simulink model "Furnace"  (R2020a)
settings: Solver=ode15s  StartTime=0  StopTime=12000  FixedStep=0.1  MaxStep=20  RelTol=1e-08  AbsTol=1e-09
undefined symbols (not defined in the file): k, reg
libraries: simulink x9, mpclib x1
(part 1 of 3)
settings Model: SimulationMode=accelerator  Creator=elisam  LastModifiedBy=jorn
settings SolverCC: MaxConsecutiveZCs=10000  ZeroCrossAlgorithm=Adaptive
settings DataIOCC: FinalStateName=ss_state_out  InitialState=ss_state  SaveFinalState=on  SaveOperatingPoint=on  SaveFormat=StructureWithTime  SaveOutput=off  DSMLogging=off  ReturnWorkspaceOutputs=off
settings OptimizationCC: BlockReduction=off  EfficientMapNaN2IntZero=off  SimCompilerOptimization=on
settings DebuggingCC: AlgebraicLoopMsg=error  ArtificialAlgebraicLoopMsg=error  UnconnectedInputMsg=none  UnconnectedOutputMsg=none  UnconnectedLineMsg=none  PregeneratedLibrarySubsystemCodeDiagnostic=none  ArithmeticOperatorsInVariantConditions=warning
settings HardwareCC: TargetBitPerLong=64  TargetBitPerPointer=64  TargetBitPerSizeT=64  TargetBitPerPtrDiffT=64  TargetLongLongMode=on  TargetIntDivRoundTo=Zero  TargetEndianess=LittleEndian  TargetWordSize=64  TargetHWDeviceType=MATLAB Host  ProdEqTarget=off
settings SFSimCC: SimUseLocalCustomCode=off  CustomCodeUndefinedFunction=UseInterfaceOnly
settings CodeAppCC: MaxIdLength=128
settings GRTTargetCC: TargetLangStandard=C89/C90 (ANSI)  CombineOutputUpdateFcns=off  GRTInterface=on

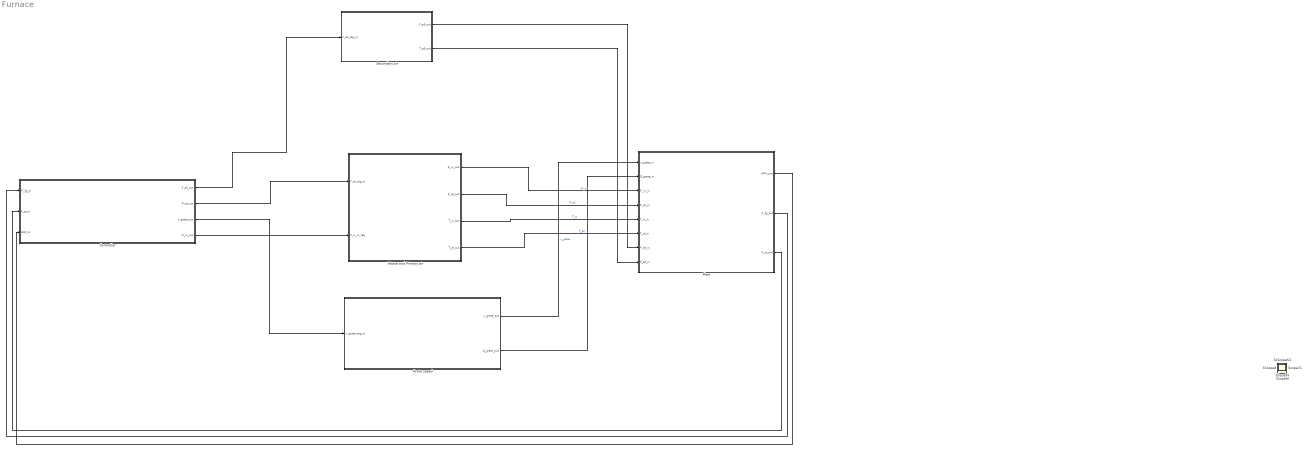
== system Furnace ==
  Controller : Subsystem
  Grate speed : Subsystem
  Plant : Subsystem
  Secondary air : Subsystem
      mask Display: image('airflow.jpeg');
  Waste and Primary air : Subsystem
      mask Display: image('waste_in.jpg');
  Scope{,1..15,17..21} (21 alike) : Scope
  wires:
  Controller/1(F_aII_out) -> Secondary air/1(F_aII_reg_in)
  Controller/2(Fi_aI_out) -> Waste and Primary air/1("F_aI_reg_in ")
  Controller/3(v_grate_out) -> Grate speed/1(v_grate_reg_in)
  Controller/4(Fi_w_out) -> Waste and Primary air/2(F_w_in_reg)
  Grate speed/1(v_grate_out) -> Plant/1(v_grate_in)  "v_grate"
  Grate speed/2(Q_grate_out) -> Plant/2(Q_grate_in)
  Plant/2(F_fg_out) -> Controller/1(Fi_fg_in)
  Plant/3(F_st_out) -> Controller/2(F_st_in)
  Waste and Primary air/1(Fi_w_out) -> Plant/3(Fi_w_in)  "Fi_w"
  Waste and Primary air/2(Fi_aI_out) -> Plant/4(Fi_aI_in)  "Fi_aI"
  Waste and Primary air/3(T_w_out) -> Plant/5(T_w_in)  "T_w"
  Waste and Primary air/4(T_aI_out) -> Plant/6(T_aI_in)  "T_aI"
  Secondary air/1(F_aII_out) -> Plant/7(F_aII_in)
  Secondary air/2(T_aII_out) -> Plant/8(T_aII_in)
  Plant/1(HHV_out) -> Controller/3(HHV_in)

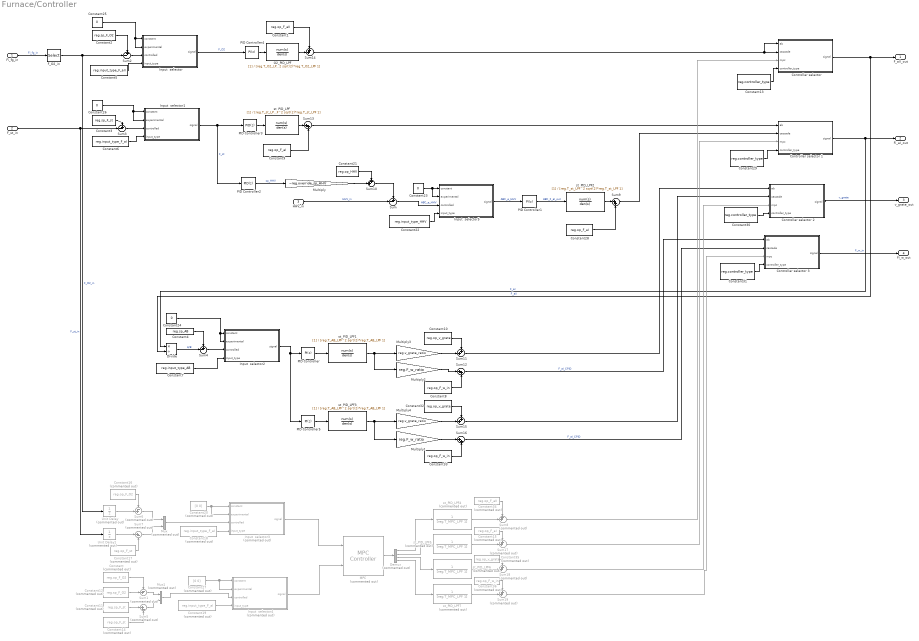
== system Furnace/Controller ==
  Fi_fg_in : Inport
  F_st_in : Inport  Port=2
  HHV_in : Inport  Port=3
  Constant : Constant  Commented=on  Value=reg.op_F_O2
  Constant1 : Constant  Value=reg.op_F_aII
  Constant10 : Constant  Value=reg.op_v_grate
  Constant11 : Constant  Commented=on  Value=reg.sp_F_st
  Constant12 : Constant  Commented=on  Value=reg.sp_F_O2
  Constant{13,29..31} (4 alike) : Constant  Value=reg.controller_type
  Constant14 : Constant  Commented=on  Value=reg.op_F_st
  Constant15 : Constant  Commented=on  Value=reg.op_F_aI
  Constant16 : Constant  Commented=on  Value=reg.op_F_O2
  Constant17 : Constant  Commented=on  Value=reg.op_F_st
  Constant18 : Constant  Commented=on  Value=reg.input_type_F_aI
  Constant19 : Constant  Commented=on  Value=reg.input_type_F_aI
  Constant2 : Constant  Value=reg.sp_F_O2
  Constant20 : Constant  Commented=on  Value=[0 0]
  Constant21 : Constant  Value=reg.op_HHV
  Constant22 : Constant  Value=reg.input_type_HHV
  Constant{23..26} (4 alike) : Constant  Value=0
  Constant27 : Constant  Commented=on  Value=[0 0]
  Constant28 : Constant  Value=reg.op_F_aI
  Constant3 : Constant  Value=reg.sp_F_st
  Constant32 : Constant  Value=reg.op_v_grate
  Constant33 : Constant  Value=reg.op_F_w_in
  Constant34 : Constant  Commented=on  Value=reg.op_F_aII
  Constant35 : Constant  Commented=on  Value=reg.op_v_grate
  Constant36 : Constant  Commented=on  Value=reg.op_F_w_in
  Constant4 : Constant  Value=reg.sp_AB
  Constant5 : Constant  Value=reg.input_type_F_aII
  Constant6 : Constant  Value=reg.input_type_F_aI
  Constant7 : Constant  Value=reg.input_type_AB
  Constant8 : Constant  Value=reg.op_F_w_in
  Constant9 : Constant  Value=reg.op_F_aI
  "Controller selector " : MATLAB Function  TreatAsAtomicUnit=on
  Controller selector 1 : MATLAB Function  TreatAsAtomicUnit=on
  Controller selector 2 : MATLAB Function  TreatAsAtomicUnit=on
  Controller selector 3 : MATLAB Function  TreatAsAtomicUnit=on
  Demux : Demux  Commented=on
  Divide : Product  Inputs=*/  OutMin=[-100]  OutMax=[100]
  F_O2_in : Selector  InputPortWidth=12  IndexOptions=Index vector (dialog)  Indices=[4]  OutputSizes=1
  Input  selector : MATLAB Function  TreatAsAtomicUnit=on
  Input  selector1 : MATLAB Function  TreatAsAtomicUnit=on
  Input  selector2 : MATLAB Function  TreatAsAtomicUnit=on
  Input  selector3 : MATLAB Function  Commented=on  TreatAsAtomicUnit=on
  Input  selector4 : MATLAB Function  Commented=on  TreatAsAtomicUnit=on
  Input  selector5 : MATLAB Function  TreatAsAtomicUnit=on
  MPC : mpclib/MPC Controller  Commented=on  SCDEnableBlockLinearizationSpecification=on  mpcobj=lmpc  is_multiple=0  enable_value=0  return_u0=off  updateMPCinCallerWorkspace=on  md_inport=off  mv_inport=off  uref_inport=off  return_cost=off  return_mvseq=off  return_qpstatus=off  return_xseq=off  return_state=off  return_ovseq=off  state_inport=off  umin_inport=off  umax_inport=off  ymin_inport=off  ymax_inport=off  cc_inport=off  ywt_inport=off  uwt_inport=off  duwt_inport=off  rhoeps_inport=off  pm_inport=off  MaximumP=10  HorizonChoice=FixedHorizon  n_ts=20  n_p=50  n_mv=4  n_md=0  n_ud=0  n_mo=2  n_uo=0  BlockDataType=double  SampleTimeInherited=off  switch_inport=off
  Multiply : Gain  Gain=~reg.override_sp_HHV
  Multiply1 : Gain  Gain=reg.F_w_ratio
  Multiply2 : Gain  Gain=reg.F_w_ratio
  Multiply3 : Gain  Gain=reg.v_grate_ratio
  Multiply4 : Gain  Gain=reg.v_grate_ratio
  Mux : Mux  Commented=on  Inputs=2
  Mux1 : Mux  Commented=on  Inputs=2
  O2_PID_LPF : TransferFcn  Denominator=[reg.T_O2_LPF^2 sqrt(2)*reg.T_O2_LPF 1]
  PID Controller : simulink/Continuous/PID Controller  Controller=PI  Form=Parallel  TimeDomain=Discrete-time  UseExternalTs=off  SampleTime=1  IntegratorMethod=Forward Euler  FilterMethod=Forward Euler  ControllerParametersSource=internal  P=reg.Kp_AB  I=reg.Ki_AB  D=0  UseFilter=on  N=100  TunerSelectOption=Transfer Function Based (PID Tuner App)  InitialConditionSource=internal  InitialConditionForIntegrator=0  InitialConditionForFilter=0  DifferentiatorICPrevScaledInput=0  ExternalReset=none  TrackingMode=off  Kt=1  LimitOutput=off  UpperSaturationLimit=inf  LowerSaturationLimit=-inf  LinearizeAsGain=on  AntiWindupMode=none  Kb=1  POutMin=[]  POutMax=[]  IOutMin=[]  IOutMax=[]  DOutMin=[]  DOutMax=[]  NOutMin=[]  NOutMax=[]  SumOutMin=[]  SumOutMax=[]  SaturationOutMin=[]  SaturationOutMax=[]  PParamMin=[]  PParamMax=[]  IParamMin=[]  IParamMax=[]  DParamMin=[]  DParamMax=[]  NParamMin=[]  NParamMax=[]  KbParamMin=[]  KbParamMax=[]  KtParamMin=[]  KtParamMax=[]  KbOutMin=[]  KbOutMax=[]  KtOutMin=[]  KtOutMax=[]  IntegratorOutMin=[]  IntegratorOutMax=[]  FilterOutMin=[]  FilterOutMax=[]  SumI1OutMin=[]  SumI1OutMax=[]  SumI2OutMin=[]  SumI2OutMax=[]  SumI3OutMin=[]  SumI3OutMax=[]  SumI4OutMin=[]  SumI4OutMax=[]  SumDOutMin=[]  SumDOutMax=[]  DifferentiatorOutMin=[]  DifferentiatorOutMax=[]  FilterDiffOutCoefMin=[]  FilterDiffOutCoefMax=[]  ReciprocalOutMin=[]  ReciprocalOutMax=[]  SumDenOutMin=[]  SumDenOutMax=[]  SumNumOutMin=[]  SumNumOutMax=[]  DivideOutMin=[]  DivideOutMax=[]  UdiffTsProdOutMin=[]  UdiffTsProdOutMax=[]  NTsProdOutMin=[]  NTsProdOutMax=[]  UintegralTsProdOutMin=[]  UintegralTsProdOutMax=[]  UngainTsProdOutMin=[]  UngainTsProdOutMax=[]  IntegratorContinuousStateAttributes=''  IntegratorStateMustResolveToSignalObject=off  IntegratorRTWStateStorageClass=Auto  FilterContinuousStateAttributes=''  FilterStateMustResolveToSignalObject=off  FilterRTWStateStorageClass=Auto  ParallelPVariant=InternalParameters  IdealPVariant=Disabled  IVariant=InternalParameters  DVariant=Disabled  IntegratorVariant=Discrete  SatVariant=Disabled  AWVariant=Passthrough  PCopyVariant=Disabled  TRVariant=Disabled  FdbkBlocksVariant=Forward  IdealPFdbkVariant=Disabled  SatFdbkVariant=Disabled  DerivativeFilterVariant=Disabled  NVariant=Disabled  NCopyVariant=Disabled_SignalSpec  FilterICVariant=Disabled  IntegratorICVariant=InternalICs  ExternalResetVariant=Disabled  TRSumVariant=Passthrough  SumFdbkVariant=Disabled  SumVariant=Sum_PI  TsampFilterVariant=InternalTs  TsampNgainVariant=Passthrough  TsampIntegralVariant=Passthrough
  PID Controller1 : simulink/Continuous/PID Controller  Controller=PI  Form=Parallel  TimeDomain=Discrete-time  UseExternalTs=off  SampleTime=1  IntegratorMethod=Forward Euler  FilterMethod=Forward Euler  ControllerParametersSource=internal  P=reg.Kp_HHV  I=reg.Ki_HHV  D=0  UseFilter=on  N=100  TunerSelectOption=Transfer Function Based (PID Tuner App)  InitialConditionSource=internal  InitialConditionForIntegrator=0  InitialConditionForFilter=0  DifferentiatorICPrevScaledInput=0  ExternalReset=none  TrackingMode=off  Kt=1  LimitOutput=off  UpperSaturationLimit=inf  LowerSaturationLimit=-inf  LinearizeAsGain=on  AntiWindupMode=none  Kb=1  POutMin=[]  POutMax=[]  IOutMin=[]  IOutMax=[]  DOutMin=[]  DOutMax=[]  NOutMin=[]  NOutMax=[]  SumOutMin=[]  SumOutMax=[]  SaturationOutMin=[]  SaturationOutMax=[]  PParamMin=[]  PParamMax=[]  IParamMin=[]  IParamMax=[]  DParamMin=[]  DParamMax=[]  NParamMin=[]  NParamMax=[]  KbParamMin=[]  KbParamMax=[]  KtParamMin=[]  KtParamMax=[]  KbOutMin=[]  KbOutMax=[]  KtOutMin=[]  KtOutMax=[]  IntegratorOutMin=[]  IntegratorOutMax=[]  FilterOutMin=[]  FilterOutMax=[]  SumI1OutMin=[]  SumI1OutMax=[]  SumI2OutMin=[]  SumI2OutMax=[]  SumI3OutMin=[]  SumI3OutMax=[]  SumI4OutMin=[]  SumI4OutMax=[]  SumDOutMin=[]  SumDOutMax=[]  DifferentiatorOutMin=[]  DifferentiatorOutMax=[]  FilterDiffOutCoefMin=[]  FilterDiffOutCoefMax=[]  ReciprocalOutMin=[]  ReciprocalOutMax=[]  SumDenOutMin=[]  SumDenOutMax=[]  SumNumOutMin=[]  SumNumOutMax=[]  DivideOutMin=[]  DivideOutMax=[]  UdiffTsProdOutMin=[]  UdiffTsProdOutMax=[]  NTsProdOutMin=[]  NTsProdOutMax=[]  UintegralTsProdOutMin=[]  UintegralTsProdOutMax=[]  UngainTsProdOutMin=[]  UngainTsProdOutMax=[]  IntegratorContinuousStateAttributes=''  IntegratorStateMustResolveToSignalObject=off  IntegratorRTWStateStorageClass=Auto  FilterContinuousStateAttributes=''  FilterStateMustResolveToSignalObject=off  FilterRTWStateStorageClass=Auto  ParallelPVariant=InternalParameters  IdealPVariant=Disabled  IVariant=InternalParameters  DVariant=Disabled  IntegratorVariant=Discrete  SatVariant=Disabled  AWVariant=Passthrough  PCopyVariant=Disabled  TRVariant=Disabled  FdbkBlocksVariant=Forward  IdealPFdbkVariant=Disabled  SatFdbkVariant=Disabled  DerivativeFilterVariant=Disabled  NVariant=Disabled  NCopyVariant=Disabled_SignalSpec  FilterICVariant=Disabled  IntegratorICVariant=InternalICs  ExternalResetVariant=Disabled  TRSumVariant=Passthrough  SumFdbkVariant=Disabled  SumVariant=Sum_PI  TsampFilterVariant=InternalTs  TsampNgainVariant=Passthrough  TsampIntegralVariant=Passthrough
  PID Controller2 : simulink/Continuous/PID Controller  Controller=PID  Form=Parallel  TimeDomain=Discrete-time  UseExternalTs=off  SampleTime=1  IntegratorMethod=Forward Euler  FilterMethod=Forward Euler  ControllerParametersSource=internal  P=reg.Kp_st_HHV  I=reg.Ki_st_HHV  D=reg.Kd_st_HHV  UseFilter=on  N=100  TunerSelectOption=Transfer Function Based (PID Tuner App)  InitialConditionSource=internal  InitialConditionForIntegrator=0.001  InitialConditionForFilter=0  DifferentiatorICPrevScaledInput=0  ExternalReset=none  TrackingMode=off  Kt=1  LimitOutput=off  UpperSaturationLimit=inf  LowerSaturationLimit=1  LinearizeAsGain=on  AntiWindupMode=none  Kb=1  POutMin=[]  POutMax=[]  IOutMin=[]  IOutMax=[]  DOutMin=[]  DOutMax=[]  NOutMin=[]  NOutMax=[]  SumOutMin=[]  SumOutMax=[]  SaturationOutMin=[]  SaturationOutMax=[]  PParamMin=[]  PParamMax=[]  IParamMin=[]  IParamMax=[]  DParamMin=[]  DParamMax=[]  NParamMin=[]  NParamMax=[]  KbParamMin=[]  KbParamMax=[]  KtParamMin=[]  KtParamMax=[]  KbOutMin=[]  KbOutMax=[]  KtOutMin=[]  KtOutMax=[]  IntegratorOutMin=[]  IntegratorOutMax=[]  FilterOutMin=[]  FilterOutMax=[]  SumI1OutMin=[]  SumI1OutMax=[]  SumI2OutMin=[]  SumI2OutMax=[]  SumI3OutMin=[]  SumI3OutMax=[]  SumI4OutMin=[]  SumI4OutMax=[]  SumDOutMin=[]  SumDOutMax=[]  DifferentiatorOutMin=[]  DifferentiatorOutMax=[]  FilterDiffOutCoefMin=[]  FilterDiffOutCoefMax=[]  ReciprocalOutMin=[]  ReciprocalOutMax=[]  SumDenOutMin=[]  SumDenOutMax=[]  SumNumOutMin=[]  SumNumOutMax=[]  DivideOutMin=[]  DivideOutMax=[]  UdiffTsProdOutMin=[]  UdiffTsProdOutMax=[]  NTsProdOutMin=[]  NTsProdOutMax=[]  UintegralTsProdOutMin=[]  UintegralTsProdOutMax=[]  UngainTsProdOutMin=[]  UngainTsProdOutMax=[]  IntegratorContinuousStateAttributes='F_st'  IntegratorStateMustResolveToSignalObject=off  IntegratorRTWStateStorageClass=Auto  FilterContinuousStateAttributes=''  FilterStateMustResolveToSignalObject=off  FilterRTWStateStorageClass=Auto  ParallelPVariant=InternalParameters  IdealPVariant=Disabled  IVariant=InternalParameters  DVariant=InternalParameters  IntegratorVariant=Discrete  SatVariant=Disabled  AWVariant=Passthrough  PCopyVariant=Disabled  TRVariant=Disabled  FdbkBlocksVariant=Forward  IdealPFdbkVariant=Disabled  SatFdbkVariant=Disabled  DerivativeFilterVariant=ForwardEulerFilter  NVariant=InternalParameters  NCopyVariant=Disabled  FilterICVariant=InternalICsFilter  IntegratorICVariant=InternalICs  ExternalResetVariant=Disabled  TRSumVariant=Passthrough  SumFdbkVariant=Disabled  SumVariant=Sum_PID  TsampFilterVariant=InternalTs  TsampNgainVariant=Passthrough  TsampIntegralVariant=Passthrough
  PID Controller3 : simulink/Continuous/PID Controller  Controller=PID  Form=Parallel  TimeDomain=Discrete-time  UseExternalTs=off  SampleTime=1  IntegratorMethod=Forward Euler  FilterMethod=Forward Euler  ControllerParametersSource=internal  P=reg.Kp_st  I=reg.Ki_st  D=reg.Kd_st  UseFilter=on  N=100  TunerSelectOption=Transfer Function Based (PID Tuner App)  InitialConditionSource=internal  InitialConditionForIntegrator=0  InitialConditionForFilter=0  DifferentiatorICPrevScaledInput=0  ExternalReset=none  TrackingMode=off  Kt=1  LimitOutput=off  UpperSaturationLimit=inf  LowerSaturationLimit=1  LinearizeAsGain=on  AntiWindupMode=none  Kb=1  POutMin=[]  POutMax=[]  IOutMin=[]  IOutMax=[]  DOutMin=[]  DOutMax=[]  NOutMin=[]  NOutMax=[]  SumOutMin=[]  SumOutMax=[]  SaturationOutMin=[]  SaturationOutMax=[]  PParamMin=[]  PParamMax=[]  IParamMin=[]  IParamMax=[]  DParamMin=[]  DParamMax=[]  NParamMin=[]  NParamMax=[]  KbParamMin=[]  KbParamMax=[]  KtParamMin=[]  KtParamMax=[]  KbOutMin=[]  KbOutMax=[]  KtOutMin=[]  KtOutMax=[]  IntegratorOutMin=[]  IntegratorOutMax=[]  FilterOutMin=[]  FilterOutMax=[]  SumI1OutMin=[]  SumI1OutMax=[]  SumI2OutMin=[]  SumI2OutMax=[]  SumI3OutMin=[]  SumI3OutMax=[]  SumI4OutMin=[]  SumI4OutMax=[]  SumDOutMin=[]  SumDOutMax=[]  DifferentiatorOutMin=[]  DifferentiatorOutMax=[]  FilterDiffOutCoefMin=[]  FilterDiffOutCoefMax=[]  ReciprocalOutMin=[]  ReciprocalOutMax=[]  SumDenOutMin=[]  SumDenOutMax=[]  SumNumOutMin=[]  SumNumOutMax=[]  DivideOutMin=[]  DivideOutMax=[]  UdiffTsProdOutMin=[]  UdiffTsProdOutMax=[]  NTsProdOutMin=[]  NTsProdOutMax=[]  UintegralTsProdOutMin=[]  UintegralTsProdOutMax=[]  UngainTsProdOutMin=[]  UngainTsProdOutMax=[]  IntegratorContinuousStateAttributes='F_st'  IntegratorStateMustResolveToSignalObject=off  IntegratorRTWStateStorageClass=Auto  FilterContinuousStateAttributes=''  FilterStateMustResolveToSignalObject=off  FilterRTWStateStorageClass=Auto  ParallelPVariant=InternalParameters  IdealPVariant=Disabled  IVariant=InternalParameters  DVariant=InternalParameters  IntegratorVariant=Discrete  SatVariant=Disabled  AWVariant=Passthrough  PCopyVariant=Disabled  TRVariant=Disabled  FdbkBlocksVariant=Forward  IdealPFdbkVariant=Disabled  SatFdbkVariant=Disabled  DerivativeFilterVariant=ForwardEulerFilter  NVariant=InternalParameters  NCopyVariant=Disabled  FilterICVariant=InternalICsFilter  IntegratorICVariant=InternalICs  ExternalResetVariant=Disabled  TRSumVariant=Passthrough  SumFdbkVariant=Disabled  SumVariant=Sum_PID  TsampFilterVariant=InternalTs  TsampNgainVariant=Passthrough  TsampIntegralVariant=Passthrough
  PID Controller4 : simulink/Continuous/PID Controller  Controller=PI  Form=Parallel  TimeDomain=Discrete-time  UseExternalTs=off  SampleTime=1  IntegratorMethod=Forward Euler  FilterMethod=Forward Euler  ControllerParametersSource=internal  P=reg.Kp_O2  I=reg.Ki_O2  D=0  UseFilter=on  N=100  TunerSelectOption=Transfer Function Based (PID Tuner App)  InitialConditionSource=internal  InitialConditionForIntegrator=0.001  InitialConditionForFilter=0  DifferentiatorICPrevScaledInput=0  ExternalReset=none  TrackingMode=off  Kt=1  LimitOutput=off  UpperSaturationLimit=inf  LowerSaturationLimit=1  LinearizeAsGain=on  AntiWindupMode=none  Kb=1  POutMin=[]  POutMax=[]  IOutMin=[]  IOutMax=[]  DOutMin=[]  DOutMax=[]  NOutMin=[]  NOutMax=[]  SumOutMin=[]  SumOutMax=[]  SaturationOutMin=[]  SaturationOutMax=[]  PParamMin=[]  PParamMax=[]  IParamMin=[]  IParamMax=[]  DParamMin=[]  DParamMax=[]  NParamMin=[]  NParamMax=[]  KbParamMin=[]  KbParamMax=[]  KtParamMin=[]  KtParamMax=[]  KbOutMin=[]  KbOutMax=[]  KtOutMin=[]  KtOutMax=[]  IntegratorOutMin=[]  IntegratorOutMax=[]  FilterOutMin=[]  FilterOutMax=[]  SumI1OutMin=[]  SumI1OutMax=[]  SumI2OutMin=[]  SumI2OutMax=[]  SumI3OutMin=[]  SumI3OutMax=[]  SumI4OutMin=[]  SumI4OutMax=[]  SumDOutMin=[]  SumDOutMax=[]  DifferentiatorOutMin=[]  DifferentiatorOutMax=[]  FilterDiffOutCoefMin=[]  FilterDiffOutCoefMax=[]  ReciprocalOutMin=[]  ReciprocalOutMax=[]  SumDenOutMin=[]  SumDenOutMax=[]  SumNumOutMin=[]  SumNumOutMax=[]  DivideOutMin=[]  DivideOutMax=[]  UdiffTsProdOutMin=[]  UdiffTsProdOutMax=[]  NTsProdOutMin=[]  NTsProdOutMax=[]  UintegralTsProdOutMin=[]  UintegralTsProdOutMax=[]  UngainTsProdOutMin=[]  UngainTsProdOutMax=[]  IntegratorContinuousStateAttributes='F_st'  IntegratorStateMustResolveToSignalObject=off  IntegratorRTWStateStorageClass=Auto  FilterContinuousStateAttributes=''  FilterStateMustResolveToSignalObject=off  FilterRTWStateStorageClass=Auto  ParallelPVariant=InternalParameters  IdealPVariant=Disabled  IVariant=InternalParameters  DVariant=Disabled  IntegratorVariant=Discrete  SatVariant=Disabled  AWVariant=Passthrough  PCopyVariant=Disabled  TRVariant=Disabled  FdbkBlocksVariant=Forward  IdealPFdbkVariant=Disabled  SatFdbkVariant=Disabled  DerivativeFilterVariant=Disabled  NVariant=Disabled  NCopyVariant=Disabled_SignalSpec  FilterICVariant=Disabled  IntegratorICVariant=InternalICs  ExternalResetVariant=Disabled  TRSumVariant=Passthrough  SumFdbkVariant=Disabled  SumVariant=Sum_PI  TsampFilterVariant=InternalTs  TsampNgainVariant=Passthrough  TsampIntegralVariant=Passthrough
  PID Controller5 : simulink/Continuous/PID Controller  Controller=PI  Form=Parallel  TimeDomain=Discrete-time  UseExternalTs=off  SampleTime=1  IntegratorMethod=Forward Euler  FilterMethod=Forward Euler  ControllerParametersSource=internal  P=reg.Kp_AB_HHV  I=reg.Ki_AB_HHV  D=0  UseFilter=on  N=100  TunerSelectOption=Transfer Function Based (PID Tuner App)  InitialConditionSource=internal  InitialConditionForIntegrator=0  InitialConditionForFilter=0  DifferentiatorICPrevScaledInput=0  ExternalReset=none  TrackingMode=off  Kt=1  LimitOutput=off  UpperSaturationLimit=inf  LowerSaturationLimit=-inf  LinearizeAsGain=on  AntiWindupMode=none  Kb=1  POutMin=[]  POutMax=[]  IOutMin=[]  IOutMax=[]  DOutMin=[]  DOutMax=[]  NOutMin=[]  NOutMax=[]  SumOutMin=[]  SumOutMax=[]  SaturationOutMin=[]  SaturationOutMax=[]  PParamMin=[]  PParamMax=[]  IParamMin=[]  IParamMax=[]  DParamMin=[]  DParamMax=[]  NParamMin=[]  NParamMax=[]  KbParamMin=[]  KbParamMax=[]  KtParamMin=[]  KtParamMax=[]  KbOutMin=[]  KbOutMax=[]  KtOutMin=[]  KtOutMax=[]  IntegratorOutMin=[]  IntegratorOutMax=[]  FilterOutMin=[]  FilterOutMax=[]  SumI1OutMin=[]  SumI1OutMax=[]  SumI2OutMin=[]  SumI2OutMax=[]  SumI3OutMin=[]  SumI3OutMax=[]  SumI4OutMin=[]  SumI4OutMax=[]  SumDOutMin=[]  SumDOutMax=[]  DifferentiatorOutMin=[]  DifferentiatorOutMax=[]  FilterDiffOutCoefMin=[]  FilterDiffOutCoefMax=[]  ReciprocalOutMin=[]  ReciprocalOutMax=[]  SumDenOutMin=[]  SumDenOutMax=[]  SumNumOutMin=[]  SumNumOutMax=[]  DivideOutMin=[]  DivideOutMax=[]  UdiffTsProdOutMin=[]  UdiffTsProdOutMax=[]  NTsProdOutMin=[]  NTsProdOutMax=[]  UintegralTsProdOutMin=[]  UintegralTsProdOutMax=[]  UngainTsProdOutMin=[]  UngainTsProdOutMax=[]  IntegratorContinuousStateAttributes=''  IntegratorStateMustResolveToSignalObject=off  IntegratorRTWStateStorageClass=Auto  FilterContinuousStateAttributes=''  FilterStateMustResolveToSignalObject=off  FilterRTWStateStorageClass=Auto  ParallelPVariant=InternalParameters  IdealPVariant=Disabled  IVariant=InternalParameters  DVariant=Disabled  IntegratorVariant=Discrete  SatVariant=Disabled  AWVariant=Passthrough  PCopyVariant=Disabled  TRVariant=Disabled  FdbkBlocksVariant=Forward  IdealPFdbkVariant=Disabled  SatFdbkVariant=Disabled  DerivativeFilterVariant=Disabled  NVariant=Disabled  NCopyVariant=Disabled_SignalSpec  FilterICVariant=Disabled  IntegratorICVariant=InternalICs  ExternalResetVariant=Disabled  TRSumVariant=Passthrough  SumFdbkVariant=Disabled  SumVariant=Sum_PI  TsampFilterVariant=InternalTs  TsampNgainVariant=Passthrough  TsampIntegralVariant=Passthrough
  Sum{,2..4} (4 alike) : Sum  Inputs=+-|
  Sum1 : Sum  Commented=on  Inputs=-+|
  Sum{10..11,14..15} (4 alike) : Sum  Inputs=++|
  Sum{9,12..13,16} (4 alike) : Sum  Inputs=|++
  Sum{8,17..19} (4 alike) : Sum  Commented=on  Inputs=++|
  Sum5 : Sum  Commented=on  Inputs=|+-
  Sum6 : Sum  Commented=on  Inputs=-+|
  Sum7 : Sum  Commented=on  Inputs=|+-
  Unit Delay : UnitDelay  Commented=on  HasFrameUpgradeWarning=on
  Unit Delay1 : UnitDelay  Commented=on  HasFrameUpgradeWarning=on
  st_PID_LPF : TransferFcn  Denominator=[reg.T_st_LPF^2 sqrt(2)*reg.T_st_LPF 1]
  st_PID_LPF1 : TransferFcn  Denominator=[reg.T_AB_LPF^2 sqrt(2)*reg.T_AB_LPF 1]
  st_PID_LPF2 : TransferFcn  Denominator=[reg.T_st_LPF^2 sqrt(2)*reg.T_st_LPF 1]
  st_PID_LPF3 : TransferFcn  Denominator=[reg.T_AB_LPF^2 sqrt(2)*reg.T_AB_LPF 1]
  st_PID_LPF{4..7} (4 alike) : TransferFcn  Commented=on  Denominator=[reg.T_MPC_LPF 1]
  F_aII_out : Outport  VectorParamsAs1DForOutWhenUnconnected=off
  Fi_aI_out : Outport  Port=2  VectorParamsAs1DForOutWhenUnconnected=off
  v_grate_out : Outport  Port=3  VectorParamsAs1DForOutWhenUnconnected=off
  Fi_w_out : Outport  Port=4  VectorParamsAs1DForOutWhenUnconnected=off
  wires:
  Input  selector/1(signal) -> PID Controller4/1  "F_O2"
  Constant7/1 -> Input  selector2/4(input_type)
  Constant5/1 -> Input  selector/4(input_type)
  Constant4/1 -> Sum4/1
  Fi_fg_in/1 -> F_O2_in/1  "Fi_fg_in"
  Constant2/1 -> Sum2/1
  F_st_in/1 -> Unit Delay1/1, Sum3/2  "F_st_in"
  Constant3/1 -> Sum3/1
  F_O2_in/1 -> Unit Delay/1, Sum2/2  "F_O2_in"
  PID Controller4/1 -> O2_PID_LPF/1
  Sum14/1 -> "Controller selector "/1(ab), "Controller selector "/2(cascade)
  PID Controller3/1 -> st_PID_LPF/1
  Sum13/1 -> Controller selector 1/1(ab)
  Constant8/1 -> Sum12/2
  PID Controller/1 -> st_PID_LPF1/1
  Sum11/1 -> Controller selector 2/1(ab)
  Multiply2/1 -> Sum12/1
  Constant10/1 -> Sum11/1
  st_PID_LPF/1 -> Sum13/1
  st_PID_LPF1/1 -> Multiply2/1, Multiply3/1
  Demux/1 -> st_PID_LPF4/1
  Demux/2 -> st_PID_LPF5/1
  Demux/3 -> st_PID_LPF6/1
  Demux/4 -> st_PID_LPF7/1
  "Controller selector "/1(signal) -> Divide/2, F_aII_out/1  "F_aII"
  Controller selector 1/1(signal) -> Divide/1, Fi_aI_out/1  "F_aI"
  Controller selector 2/1(signal) -> v_grate_out/1  "v_grate"
  Controller selector 3/1(signal) -> Fi_w_out/1  "F_w_in"
  Constant12/1 -> Sum1/2
  Constant/1 -> Sum1/1
  Constant11/1 -> Sum5/1
  Constant14/1 -> Sum5/2
  Sum5/1 -> Mux1/2
  MPC/1 -> Demux/1
  Sum7/1 -> Mux/2
  Constant16/1 -> Sum6/1
  Constant17/1 -> Sum7/2
  Input  selector3/1(signal) -> MPC/1
  Mux/1 -> Input  selector3/3(controlled)
  Constant18/1 -> Input  selector3/4(input_type)
  Constant19/1 -> Input  selector4/4(input_type)
  Mux1/1 -> Input  selector4/3(controlled)
  Input  selector4/1(signal) -> MPC/2
  Constant20/1 -> Input  selector3/2(experimental), Input  selector3/1(constant)
  HHV_in/1 -> Sum/2  "HHV_in"
  Input  selector5/1(signal) -> PID Controller1/1  "ABC_e_HHV"
  Constant22/1 -> Input  selector5/4(input_type)
  Sum/1 -> Input  selector5/3(controlled)  "ABC_e_HHV"
  Constant23/1 -> Input  selector5/2(experimental), Input  selector5/1(constant)
  Divide/1 -> Sum4/2  "A/B"
  Sum4/1 -> Input  selector2/3(controlled)
  Input  selector2/1(signal) -> PID Controller5/1, PID Controller/1
  Constant24/1 -> Input  selector2/2(experimental), Input  selector2/1(constant)
  Sum2/1 -> Input  selector/3(controlled)
  Constant25/1 -> Input  selector/2(experimental), Input  selector/1(constant)
  Sum3/1 -> Input  selector1/3(controlled)
  Constant6/1 -> Input  selector1/4(input_type)
  Constant26/1 -> Input  selector1/2(experimental), Input  selector1/1(constant)
  Input  selector1/1(signal) -> PID Controller3/1, PID Controller2/1  "F_st"
  Constant27/1 -> Input  selector4/2(experimental), Input  selector4/1(constant)
  Sum12/1 -> Controller selector 3/1(ab)  "F_aI_CPID"
  PID Controller1/1 -> st_PID_LPF2/1  "ABC_F_aI_out"
  Sum9/1 -> Controller selector 1/2(cascade)
  PID Controller2/1 -> Multiply/1  "sp_HHV"
  Multiply/1 -> Sum10/2
  Constant21/1 -> Sum10/1
  Sum10/1 -> Sum/1
  st_PID_LPF2/1 -> Sum9/1
  Sum1/1 -> Mux1/1
  Sum6/1 -> Mux/1
  Constant28/1 -> Sum9/2
  Constant9/1 -> Sum13/2
  O2_PID_LPF/1 -> Sum14/2
  Constant1/1 -> Sum14/1
  Constant13/1 -> "Controller selector "/4(controller_type)
  Constant29/1 -> Controller selector 1/4(controller_type)
  Constant30/1 -> Controller selector 2/4(controller_type)
  Constant31/1 -> Controller selector 3/4(controller_type)
  st_PID_LPF3/1 -> Multiply1/1, Multiply4/1
  PID Controller5/1 -> st_PID_LPF3/1
  Constant33/1 -> Sum16/2
  Constant32/1 -> Sum15/1
  Multiply1/1 -> Sum16/1
  Sum15/1 -> Controller selector 2/2(cascade)
  Sum16/1 -> Controller selector 3/2(cascade)  "F_aI_CPID"
  Unit Delay/1 -> Sum6/2
  Unit Delay1/1 -> Sum7/1
  st_PID_LPF4/1 -> Sum8/2
  st_PID_LPF5/1 -> Sum17/2
  st_PID_LPF6/1 -> Sum18/2
  st_PID_LPF7/1 -> Sum19/2
  Constant34/1 -> Sum8/1
  Constant15/1 -> Sum17/1
  Constant35/1 -> Sum18/1
  Constant36/1 -> Sum19/1
  Sum17/1 -> Controller selector 1/3(mpc)
  Sum8/1 -> "Controller selector "/3(mpc)
  Sum18/1 -> Controller selector 2/3(mpc)
  Sum19/1 -> Controller selector 3/3(mpc)
  Multiply3/1 -> Sum11/2
  Multiply4/1 -> Sum15/2

== system Furnace/Grate speed ==
  v_grate_reg_in : Inport
  Constant : Constant  Value=reg.const_Q_grate
  Constant1 : Constant  Value=reg.input_type_v_grate
  Constant2 : Constant  Value=reg.input_type_Q_grate
  From Workspace2 : FromWorkspace  VariableName=Q_grate
  Input selector1 : MATLAB Function  TreatAsAtomicUnit=on
  Input selector2 : MATLAB Function  TreatAsAtomicUnit=on
  const_Q_grate : Constant  Value=reg.const_Q_grate
  const_v_grate : Constant  Value=reg.const_v_grate
  v_grate : Constant  Value=k.v_grate
  v_grate_out : Outport  VectorParamsAs1DForOutWhenUnconnected=off
  Q_grate_out : Outport  Port=2  VectorParamsAs1DForOutWhenUnconnected=off
  wires:
  v_grate/1 -> Input selector1/2(experimental)
  Input selector1/1(signal) -> v_grate_out/1  "v_grate"
  Constant1/1 -> Input selector1/4(input_type)
  v_grate_reg_in/1 -> Input selector1/3(controlled)
  const_v_grate/1 -> Input selector1/1(constant)  "const_v_grate"
  const_Q_grate/1 -> Input selector2/1(constant)  "const_Q_grate"
  Constant2/1 -> Input selector2/4(input_type)
  Input selector2/1(signal) -> Q_grate_out/1  "Q_grate"
  From Workspace2/1 -> Input selector2/2(experimental)
  Constant/1 -> Input selector2/3(controlled)

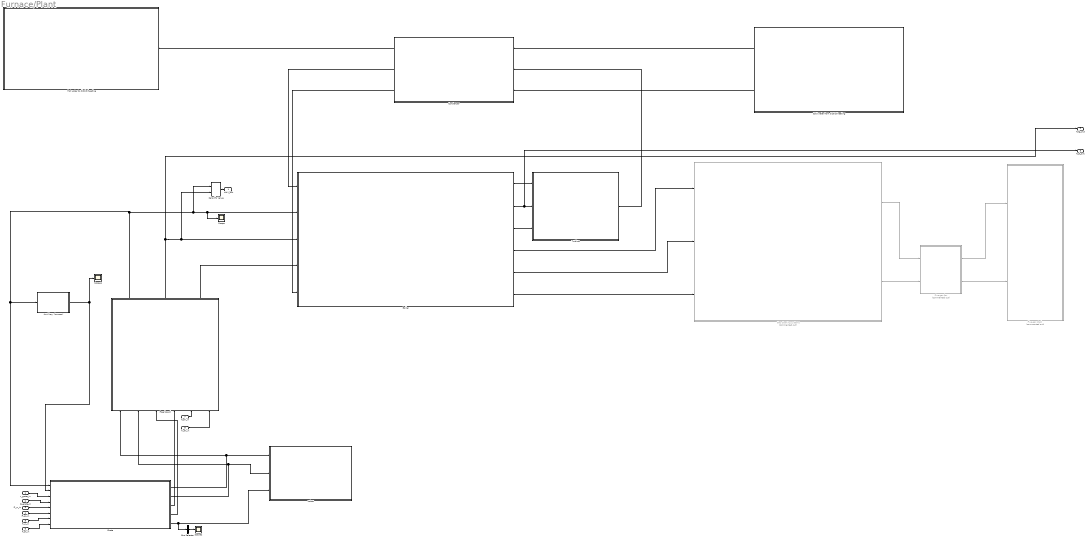
== system Furnace/Plant ==
  v_grate_in : Inport
  Q_grate_in : Inport  Port=2
  Fi_w_in : Inport  Port=3
  Fi_aI_in : Inport  Port=4
  T_w_in : Inport  Port=5
  T_aI_in : Inport  Port=6
  F_aII_in : Inport  Port=7
  T_aII_in : Inport  Port=8
  Ashes : Subsystem
      mask Display: image('ash.jpg');
  "Auxiliary \"burners\"" : Subsystem
      mask Display: image('burnerim.jpg');
  Boiler : Subsystem
      mask Display: image('Boiler.jpg');
  Bus Selector : BusSelector  OutputSignals=F_w_ash
  Calorific Value : Subsystem
  Cold water from district heating : Subsystem
      mask Display: image('fromdh.jpg');
  Condenser : Subsystem
      mask Display: image('Condenser.jpg');
  Flue-gas fan : Subsystem  Commented=on
      mask Display: image('Fan.jpg');
  Flue-gas stack : Subsystem  Commented=on
      mask Display: image('Stack.jpg');
  Free board : Subsystem
      mask Display: image('fbim.jpg');
  Gas cleaning systems : Subsystem  Commented=on
      mask Display: image('Cleaning.jpg');
  Grate : Subsystem
      settings: MinAlgLoopOccurrences=on
      mask Display: image('grateim.jpg');
  Hot water to district heating : Subsystem
      mask Display: image('todh.jpg');
  Scope : Scope
  Scope1 : Scope
  Scope2 : Scope
  Turbine : Subsystem
      mask Display: image('Turbine.jpg');
  HHV_out : Outport  VectorParamsAs1DForOutWhenUnconnected=off
  F_fg_out : Outport  Port=2  VectorParamsAs1DForOutWhenUnconnected=off
  F_st_out : Outport  Port=3  VectorParamsAs1DForOutWhenUnconnected=off
  wires:
  Boiler/3(p_drum) -> Turbine/3(p_drum)
  Free board/1(T_fg_out) -> Calorific Value/1(T_fg), Scope/1, Boiler/2(T_fg), Grate/1(T_rad), "Auxiliary \"burners\""/1(In1)  "T_rad"
  Turbine/1(F_turb) -> Condenser/2(F_turb)
  Grate/1(Fi_fg_from_grate) -> Ashes/1(In1), Free board/1(Fi_in)
  Q_grate_in/1 -> Grate/4(Q_grate)
  Condenser/1(T_district) -> Hot water to district heating/1(In1)
  Cold water from district heating/1(Out1) -> Condenser/1(F_district)
  Grate/2(T_w_grate) -> Ashes/2(In2), Free board/2(T_in)
  "Auxiliary \"burners\""/1(Out1) -> Scope1/1, Grate/2(Q_burners)  "Q_burners"
  Grate/4(Q_rad_fg) -> Free board/3(Q_rad)
  Free board/2(Fi_fg_to_boiler) -> F_fg_out/1, Calorific Value/2(Fi_fg), Boiler/3(F_fg)
  Flue-gas fan/1(Out1) -> Flue-gas stack/1(T_fg)
  Boiler/4(T_fg_out) -> Gas cleaning systems/1(T_fg)
  Boiler/2(F_SH) -> F_st_out/1, Turbine/2(F_SH)  "F_steam"
  Flue-gas fan/2(Out2) -> Flue-gas stack/2(Fi_fg)
  Grate/5(OutBus) -> Bus Selector/1, Ashes/3(InBus)
  Condenser/2(T_w_out) -> Boiler/1(T_fromHE)
  Gas cleaning systems/2(Fi_fg_clean) -> Flue-gas fan/2(Fi_fg)
  Boiler/1(T_SH) -> Turbine/1(T_SH)
  Free board/3(F_flyash_tot) -> Boiler/4(F_flyash)
  Grate/3(F_flyash) -> Free board/4(F_flyash_cell)
  Gas cleaning systems/1(T_fg_clean) -> Flue-gas fan/1(T_fg)
  v_grate_in/1 -> Grate/3(v_grate_in)
  Boiler/5(Fi_fg_out) -> Gas cleaning systems/2(F_fg)
  Condenser/3(F_cond) -> Boiler/5(F_ECO)
  Boiler/6(F_flyash_out) -> Gas cleaning systems/3(F_flyash)
  Cold water from district heating/2(Out2) -> Condenser/3(T_return)
  Calorific Value/1(HHV) -> HHV_out/1  "HHV"
  Fi_w_in/1 -> Grate/5(Fi_w_in)
  Fi_aI_in/1 -> Grate/6(F_aI_in)
  T_w_in/1 -> Grate/7(T_w_in)
  T_aI_in/1 -> Grate/8(T_aI_in)
  F_aII_in/1 -> Free board/5(F_aII_in)
  T_aII_in/1 -> Free board/6(T_aII_in)
  Bus Selector/1 -> Scope2/1  "<F_w_ash>"

== system Furnace/Secondary air ==
  F_aII_reg_in : Inport
  Constant : Constant  Value=reg.input_type_F_aII
  Constant2 : Constant  Value=reg.const_T_aII
  Constant3 : Constant  Value=reg.input_type_T_aII
  Flue gas fan : Subsystem
  From Workspace1 : FromWorkspace  VariableName=F_aII
  Input  selector : MATLAB Function  TreatAsAtomicUnit=on
  Input  selector1 : MATLAB Function  TreatAsAtomicUnit=on
  PID Controller : simulink/Continuous/PID Controller  Controller=PI  Form=Parallel  TimeDomain=Continuous-time  UseExternalTs=off  SampleTime=1  IntegratorMethod=Forward Euler  FilterMethod=Forward Euler  ControllerParametersSource=internal  P=reg.Kp_fan  I=reg.Ki_fan  D=0  UseFilter=on  N=100  TunerSelectOption=Transfer Function Based (PID Tuner App)  InitialConditionSource=internal  InitialConditionForIntegrator=reg.F_aII_fan_PID_int  InitialConditionForFilter=0  DifferentiatorICPrevScaledInput=0  ExternalReset=none  TrackingMode=off  Kt=1  LimitOutput=off  UpperSaturationLimit=inf  LowerSaturationLimit=-inf  LinearizeAsGain=on  AntiWindupMode=none  Kb=1  POutMin=[]  POutMax=[]  IOutMin=[]  IOutMax=[]  DOutMin=[]  DOutMax=[]  NOutMin=[]  NOutMax=[]  SumOutMin=[]  SumOutMax=[]  SaturationOutMin=[]  SaturationOutMax=[]  PParamMin=[]  PParamMax=[]  IParamMin=[]  IParamMax=[]  DParamMin=[]  DParamMax=[]  NParamMin=[]  NParamMax=[]  KbParamMin=[]  KbParamMax=[]  KtParamMin=[]  KtParamMax=[]  KbOutMin=[]  KbOutMax=[]  KtOutMin=[]  KtOutMax=[]  IntegratorOutMin=[]  IntegratorOutMax=[]  FilterOutMin=[]  FilterOutMax=[]  SumI1OutMin=[]  SumI1OutMax=[]  SumI2OutMin=[]  SumI2OutMax=[]  SumI3OutMin=[]  SumI3OutMax=[]  SumI4OutMin=[]  SumI4OutMax=[]  SumDOutMin=[]  SumDOutMax=[]  DifferentiatorOutMin=[]  DifferentiatorOutMax=[]  FilterDiffOutCoefMin=[]  FilterDiffOutCoefMax=[]  ReciprocalOutMin=[]  ReciprocalOutMax=[]  SumDenOutMin=[]  SumDenOutMax=[]  SumNumOutMin=[]  SumNumOutMax=[]  DivideOutMin=[]  DivideOutMax=[]  UdiffTsProdOutMin=[]  UdiffTsProdOutMax=[]  NTsProdOutMin=[]  NTsProdOutMax=[]  UintegralTsProdOutMin=[]  UintegralTsProdOutMax=[]  UngainTsProdOutMin=[]  UngainTsProdOutMax=[]  IntegratorContinuousStateAttributes=''  IntegratorStateMustResolveToSignalObject=off  IntegratorRTWStateStorageClass=Auto  FilterContinuousStateAttributes=''  FilterStateMustResolveToSignalObject=off  FilterRTWStateStorageClass=Auto  ParallelPVariant=InternalParameters  IdealPVariant=Disabled  IVariant=InternalParameters  DVariant=Disabled  IntegratorVariant=Continuous  SatVariant=Disabled  AWVariant=Passthrough  PCopyVariant=Disabled  TRVariant=Disabled  FdbkBlocksVariant=Forward  IdealPFdbkVariant=Disabled  SatFdbkVariant=Disabled  DerivativeFilterVariant=Disabled  NVariant=Disabled  NCopyVariant=Disabled_SignalSpec  FilterICVariant=Disabled  IntegratorICVariant=InternalICs  ExternalResetVariant=Disabled  TRSumVariant=Passthrough  SumFdbkVariant=Disabled  SumVariant=Sum_PI  TsampFilterVariant=InternalTs  TsampNgainVariant=Passthrough  TsampIntegralVariant=Passthrough
  Sum1 : Sum  Inputs=|+-
  T_aII : FromWorkspace  VariableName=T_aII
  const_F_aII : Constant  Value=reg.const_F_aII
  F_aII_out : Outport  VectorParamsAs1DForOutWhenUnconnected=off
  T_aII_out : Outport  Port=2  VectorParamsAs1DForOutWhenUnconnected=off
  tag scope: F_aII=global, T_aII=global
  wires:
  Constant2/1 -> Input  selector1/1(constant)
  T_aII/1 -> Input  selector1/2(experimental)
  F_aII_reg_in/1 -> Input  selector/3(controlled)
  From Workspace1/1 -> Input  selector/2(experimental)
  const_F_aII/1 -> Input  selector/1(constant)  "const_F_aII"
  Constant/1 -> Input  selector/4(input_type)
  Constant3/1 -> Input  selector1/4(input_type)
  Input  selector1/1(signal) -> [T_aII], T_aII_out/1
  Sum1/1 -> PID Controller/1
  PID Controller/1 -> Flue gas fan/1(PID signal)
  Input  selector/1(signal) -> Sum1/1  "F_aII"
  Flue gas fan/1(Volume flow) -> [F_aII], F_aII_out/1, Sum1/2

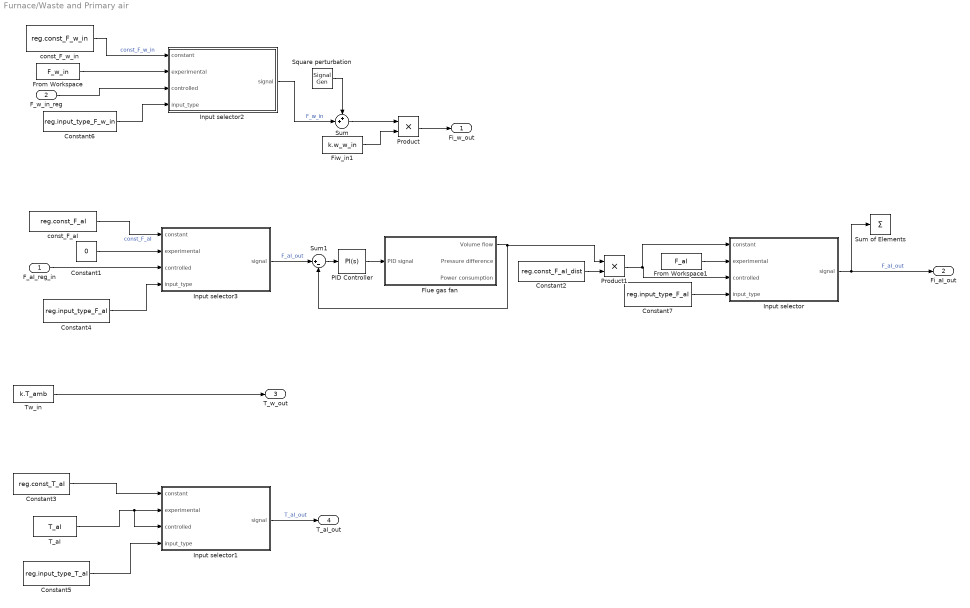
== system Furnace/Waste and Primary air ==
  "F_aI_reg_in " : Inport
  F_w_in_reg : Inport  Port=2
  Constant1 : Constant  Value=0
  Constant2 : Constant  Value=reg.const_F_aI_dist
  Constant3 : Constant  Value=reg.const_T_aI
  Constant4 : Constant  Value=reg.input_type_F_aI
  Constant5 : Constant  Value=reg.input_type_T_aI
  Constant6 : Constant  Value=reg.input_type_F_w_in
  Constant7 : Constant  Value=reg.input_type_F_aI
  Fiw_in1 : Constant  Value=k.w_w_in
  Flue gas fan : Subsystem
  From Workspace : FromWorkspace  VariableName=F_w_in
  From Workspace1 : FromWorkspace  VariableName=F_aI
  Input selector : MATLAB Function  TreatAsAtomicUnit=on
  Input selector1 : MATLAB Function  TreatAsAtomicUnit=on
  Input selector2 : MATLAB Function  TreatAsAtomicUnit=on
  Input selector3 : MATLAB Function  TreatAsAtomicUnit=on
  PID Controller : simulink/Continuous/PID Controller  Controller=PI  Form=Parallel  TimeDomain=Continuous-time  UseExternalTs=off  SampleTime=1  IntegratorMethod=Forward Euler  FilterMethod=Forward Euler  ControllerParametersSource=internal  P=reg.Kp_fan  I=reg.Ki_fan  D=0  UseFilter=on  N=100  TunerSelectOption=Transfer Function Based (PID Tuner App)  InitialConditionSource=internal  InitialConditionForIntegrator=reg.F_aI_fan_PID_int  InitialConditionForFilter=0  DifferentiatorICPrevScaledInput=0  ExternalReset=none  TrackingMode=off  Kt=1  LimitOutput=off  UpperSaturationLimit=inf  LowerSaturationLimit=-inf  LinearizeAsGain=on  AntiWindupMode=none  Kb=1  POutMin=[]  POutMax=[]  IOutMin=[]  IOutMax=[]  DOutMin=[]  DOutMax=[]  NOutMin=[]  NOutMax=[]  SumOutMin=[]  SumOutMax=[]  SaturationOutMin=[]  SaturationOutMax=[]  PParamMin=[]  PParamMax=[]  IParamMin=[]  IParamMax=[]  DParamMin=[]  DParamMax=[]  NParamMin=[]  NParamMax=[]  KbParamMin=[]  KbParamMax=[]  KtParamMin=[]  KtParamMax=[]  KbOutMin=[]  KbOutMax=[]  KtOutMin=[]  KtOutMax=[]  IntegratorOutMin=[]  IntegratorOutMax=[]  FilterOutMin=[]  FilterOutMax=[]  SumI1OutMin=[]  SumI1OutMax=[]  SumI2OutMin=[]  SumI2OutMax=[]  SumI3OutMin=[]  SumI3OutMax=[]  SumI4OutMin=[]  SumI4OutMax=[]  SumDOutMin=[]  SumDOutMax=[]  DifferentiatorOutMin=[]  DifferentiatorOutMax=[]  FilterDiffOutCoefMin=[]  FilterDiffOutCoefMax=[]  ReciprocalOutMin=[]  ReciprocalOutMax=[]  SumDenOutMin=[]  SumDenOutMax=[]  SumNumOutMin=[]  SumNumOutMax=[]  DivideOutMin=[]  DivideOutMax=[]  UdiffTsProdOutMin=[]  UdiffTsProdOutMax=[]  NTsProdOutMin=[]  NTsProdOutMax=[]  UintegralTsProdOutMin=[]  UintegralTsProdOutMax=[]  UngainTsProdOutMin=[]  UngainTsProdOutMax=[]  IntegratorContinuousStateAttributes=''  IntegratorStateMustResolveToSignalObject=off  IntegratorRTWStateStorageClass=Auto  FilterContinuousStateAttributes=''  FilterStateMustResolveToSignalObject=off  FilterRTWStateStorageClass=Auto  ParallelPVariant=InternalParameters  IdealPVariant=Disabled  IVariant=InternalParameters  DVariant=Disabled  IntegratorVariant=Continuous  SatVariant=Disabled  AWVariant=Passthrough  PCopyVariant=Disabled  TRVariant=Disabled  FdbkBlocksVariant=Forward  IdealPFdbkVariant=Disabled  SatFdbkVariant=Disabled  DerivativeFilterVariant=Disabled  NVariant=Disabled  NCopyVariant=Disabled_SignalSpec  FilterICVariant=Disabled  IntegratorICVariant=InternalICs  ExternalResetVariant=Disabled  TRSumVariant=Passthrough  SumFdbkVariant=Disabled  SumVariant=Sum_PI  TsampFilterVariant=InternalTs  TsampNgainVariant=Passthrough  TsampIntegralVariant=Passthrough
  Product : Product
  Product1 : Product
  Square perturbation : SignalGenerator  WaveForm=square  Amplitude=reg.F_w_pert_amp  Frequency=reg.F_w_pert_freq
  Sum : Sum  Inputs=++|
  Sum of Elements : Sum  Inputs=+
  Sum1 : Sum  Inputs=|+-
  T_aI : FromWorkspace  VariableName=T_aI
  Tw_in : Constant  Value=k.T_amb
  const_F_aI : Constant  Value=reg.const_F_aI
  const_F_w_in : Constant  Value=reg.const_F_w_in
  Fi_w_out : Outport  VectorParamsAs1DForOutWhenUnconnected=off
  Fi_aI_out : Outport  Port=2  VectorParamsAs1DForOutWhenUnconnected=off
  T_w_out : Outport  Port=3  VectorParamsAs1DForOutWhenUnconnected=off
  T_aI_out : Outport  Port=4  VectorParamsAs1DForOutWhenUnconnected=off
  wires:
  Tw_in/1 -> T_w_out/1
  Fiw_in1/1 -> Product/2
  From Workspace/1 -> Input selector2/2(experimental)
  Product/1 -> Fi_w_out/1
  Input selector/1(signal) -> Fi_aI_out/1, Sum of Elements/1  "F_aI_out"
  From Workspace1/1 -> Input selector/2(experimental)
  Constant4/1 -> Input selector3/4(input_type)
  Constant5/1 -> Input selector1/4(input_type)
  T_aI/1 -> Input selector1/3(controlled), Input selector1/2(experimental)
  Constant3/1 -> Input selector1/1(constant)
  Input selector1/1(signal) -> T_aI_out/1  "T_aI_out"
  Constant6/1 -> Input selector2/4(input_type)
  F_w_in_reg/1 -> Input selector2/3(controlled)
  const_F_w_in/1 -> Input selector2/1(constant)  "const_F_w_in"
  Input selector2/1(signal) -> Sum/2  "F_w_in"
  Sum/1 -> Product/1
  Square perturbation/1 -> Sum/1
  PID Controller/1 -> Flue gas fan/1(PID signal)
  Sum1/1 -> PID Controller/1
  const_F_aI/1 -> Input selector3/1(constant)  "const_F_aI"
  "F_aI_reg_in "/1 -> Input selector3/3(controlled)
  Constant1/1 -> Input selector3/2(experimental)
  Constant2/1 -> Product1/2
  Product1/1 -> Input selector/1(constant), Input selector/3(controlled)
  Constant7/1 -> Input selector/4(input_type)
  Flue gas fan/1(Volume flow) -> Sum1/2, Product1/1
  Input selector3/1(signal) -> Sum1/1  "F_aI_out"

== system Furnace/Plant/Ashes ==
  In1 : Inport
  In2 : Inport  Port=2
  In Bus Element : Inport  Port=3  PortName=InBus  Element=M_w_grate
  In Bus Element1 : Inport  Port=3  PortName=InBus  Element=M_char
  In Bus Element2 : Inport  Port=3  PortName=InBus  Element=F_w_ash
  In Bus Element3 : Inport  Port=3  PortName=InBus  Element=F_char_ash
  Flow of char ash : Display
  Flow of waste ash : Display
  Mass of char in grate : Display
  Scope1 : Scope
  Sum of Elements : Sum  Inputs=+  CollapseMode=Specified dimension
  Temperatures in grate : Display
  Waste in grate (mass) : Display
  wires:
  In Bus Element2/1 -> Flow of waste ash/1
  In Bus Element/1 -> Waste in grate (mass)/1
  In Bus Element1/1 -> Mass of char in grate/1
  In Bus Element3/1 -> Flow of char ash/1
  In1/1 -> Sum of Elements/1
  In2/1 -> Temperatures in grate/1
  Sum of Elements/1 -> Scope1/1

== system Furnace/Plant/Auxiliary "burners" ==
  In1 : Inport
  Constant : Constant  Value=0
  Constant1 : Constant  Value=850+k.T_amb
  Minus : Sum  Inputs=+-
  "Q " : Constant  Value=3.5e6
  Switch : Switch  Criteria=u2 > Threshold
  Out1 : Outport  VectorParamsAs1DForOutWhenUnconnected=off
  wires:
  Switch/1 -> Out1/1
  Constant/1 -> Switch/3
  "Q "/1 -> Switch/1
  Minus/1 -> Switch/2
  Constant1/1 -> Minus/1
  In1/1 -> Minus/2

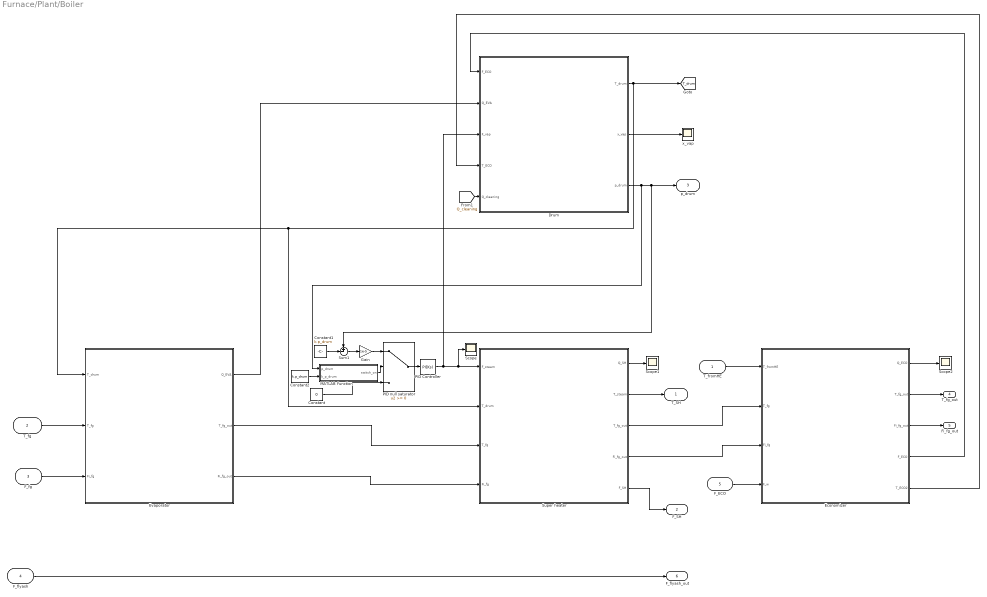
== system Furnace/Plant/Boiler ==
  T_fromHE : Inport
  T_fg : Inport  Port=2
  F_fg : Inport  Port=3
  F_flyash : Inport  Port=4
  F_ECO : Inport  Port=5
  Constant : Constant  Value=0
  Constant1 : Constant  Value=k.p_drum
  Constant2 : Constant  Value=k.p_drum
  Drum : Subsystem
      mask Display: image('Drum.jpg');
  Economizer : Subsystem
  Evaporator : Subsystem
  Gain : Gain  Gain=1e-5
  MATLAB Function : MATLAB Function  TreatAsAtomicUnit=on
  PID Controller : simulink/Continuous/PID Controller  Controller=PID  Form=Parallel  TimeDomain=Continuous-time  UseExternalTs=off  SampleTime=-1  IntegratorMethod=Forward Euler  FilterMethod=Forward Euler  ControllerParametersSource=internal  P=10  I=0  D=0  UseFilter=on  N=100  TunerSelectOption=Transfer Function Based (PID Tuner App)  InitialConditionSource=internal  InitialConditionForIntegrator=0  InitialConditionForFilter=0  DifferentiatorICPrevScaledInput=0  ExternalReset=none  TrackingMode=off  Kt=1  LimitOutput=on  UpperSaturationLimit=50  LowerSaturationLimit=0  LinearizeAsGain=on  AntiWindupMode=none  Kb=1  POutMin=[]  POutMax=[]  IOutMin=[]  IOutMax=[]  DOutMin=[]  DOutMax=[]  NOutMin=[]  NOutMax=[]  SumOutMin=[]  SumOutMax=[]  SaturationOutMin=[]  SaturationOutMax=[]  PParamMin=[]  PParamMax=[]  IParamMin=[]  IParamMax=[]  DParamMin=[]  DParamMax=[]  NParamMin=[]  NParamMax=[]  KbParamMin=[]  KbParamMax=[]  KtParamMin=[]  KtParamMax=[]  KbOutMin=[]  KbOutMax=[]  KtOutMin=[]  KtOutMax=[]  IntegratorOutMin=[]  IntegratorOutMax=[]  FilterOutMin=[]  FilterOutMax=[]  SumI1OutMin=[]  SumI1OutMax=[]  SumI2OutMin=[]  SumI2OutMax=[]  SumI3OutMin=[]  SumI3OutMax=[]  SumI4OutMin=[]  SumI4OutMax=[]  SumDOutMin=[]  SumDOutMax=[]  DifferentiatorOutMin=[]  DifferentiatorOutMax=[]  FilterDiffOutCoefMin=[]  FilterDiffOutCoefMax=[]  ReciprocalOutMin=[]  ReciprocalOutMax=[]  SumDenOutMin=[]  SumDenOutMax=[]  SumNumOutMin=[]  SumNumOutMax=[]  DivideOutMin=[]  DivideOutMax=[]  UdiffTsProdOutMin=[]  UdiffTsProdOutMax=[]  NTsProdOutMin=[]  NTsProdOutMax=[]  UintegralTsProdOutMin=[]  UintegralTsProdOutMax=[]  UngainTsProdOutMin=[]  UngainTsProdOutMax=[]  IntegratorContinuousStateAttributes=''  IntegratorStateMustResolveToSignalObject=off  IntegratorRTWStateStorageClass=Auto  FilterContinuousStateAttributes=''  FilterStateMustResolveToSignalObject=off  FilterRTWStateStorageClass=Auto  ParallelPVariant=InternalParameters  IdealPVariant=Disabled  IVariant=InternalParameters  DVariant=InternalParameters  IntegratorVariant=Continuous  SatVariant=Enabled  AWVariant=Passthrough  PCopyVariant=Disabled  TRVariant=Disabled  FdbkBlocksVariant=Forward  IdealPFdbkVariant=Disabled  SatFdbkVariant=Disabled  DerivativeFilterVariant=ContFilter  NVariant=InternalParameters  NCopyVariant=Disabled  FilterICVariant=InternalICsFilter  IntegratorICVariant=InternalICs  ExternalResetVariant=Disabled  TRSumVariant=Passthrough  SumFdbkVariant=Disabled  SumVariant=Sum_PID  TsampFilterVariant=InternalTs  TsampNgainVariant=Passthrough  TsampIntegralVariant=Passthrough
  PID null saturator : Switch
  Scope : Scope
  Scope1 : Scope
  Scope2 : Scope
  Sum1 : Sum  Inputs=+-|
  Super heater : Subsystem
  x_vap : Scope
  T_SH : Outport  VectorParamsAs1DForOutWhenUnconnected=off
  F_SH : Outport  Port=2  PortDimensions=1  VectorParamsAs1DForOutWhenUnconnected=off
  p_drum : Outport  Port=3  VectorParamsAs1DForOutWhenUnconnected=off
  T_fg_out : Outport  Port=4  VectorParamsAs1DForOutWhenUnconnected=off
  Fi_fg_out : Outport  Port=5  VectorParamsAs1DForOutWhenUnconnected=off
  F_flyash_out : Outport  Port=6  VectorParamsAs1DForOutWhenUnconnected=off
  tag scope: T_drum=global
  wires:
  Evaporator/3(Fi_fg_out) -> Super heater/4(Fi_fg)
  Super heater/4(Fi_fg_out) -> Economizer/3(Fi_fg)
  Super heater/3(T_fg_out) -> Economizer/2(T_fg)
  Evaporator/2(T_fg_out) -> Super heater/3(T_fg)
  Economizer/3(Fi_fg_out) -> Fi_fg_out/1
  F_fg/1 -> Evaporator/3(Fi_fg)
  T_fg/1 -> Evaporator/2(T_fg)
  Super heater/2(T_steam) -> T_SH/1
  Economizer/2(T_fg_out) -> T_fg_out/1
  Drum/3(p_drum) -> MATLAB Function/1(p_drum), Sum1/1, p_drum/1
  T_fromHE/1 -> Economizer/1(T_fromHE)
  Super heater/5(F_SH) -> F_SH/1
  Drum/2(x_vap) -> x_vap/1
  PID Controller/1 -> Drum/3(F_vap), Scope/1, Super heater/1(F_steam)
  Constant1/1 -> Sum1/2
  Constant/1 -> PID null saturator/3
  Sum1/1 -> Gain/1
  [Q_cleaning] -> Drum/5(Q_cleaning)
  F_flyash/1 -> F_flyash_out/1
  Super heater/1(Q_SH) -> Scope1/1
  Economizer/1(Q_ECO) -> Scope2/1
  Economizer/4(F_ECO) -> Drum/1(F_ECO)
  Evaporator/1(Q_EVA) -> Drum/2(Q_EVA)
  Economizer/5(T_ECO2) -> Drum/4(T_ECO)
  F_ECO/1 -> Economizer/4(F_w)
  PID null saturator/1 -> PID Controller/1
  Gain/1 -> PID null saturator/1
  Drum/1(T_drum) -> [T_drum], Super heater/2(T_drum), Evaporator/1(T_drum)
  MATLAB Function/1(switch_on) -> PID null saturator/2
  Constant2/1 -> MATLAB Function/2(k_p_drum)

== system Furnace/Plant/Calorific Value ==
  T_fg : Inport
  Fi_fg : Inport  Port=2
  MATLAB Function : MATLAB Function  TreatAsAtomicUnit=on
  T_amb : Constant  Value=k.T_amb
  cp_fg : Constant  Value=k.cp_fg
  HHV : Outport  VectorParamsAs1DForOutWhenUnconnected=off
  wires:
  cp_fg/1 -> MATLAB Function/3(cp_fg)
  Fi_fg/1 -> MATLAB Function/1(Fi_fg)
  T_amb/1 -> MATLAB Function/4(T_amb)
  MATLAB Function/1(HHV) -> HHV/1
  T_fg/1 -> MATLAB Function/2(T_fg)
  [F_aI] -> MATLAB Function/5(F_aI)
  [T_aI] -> MATLAB Function/6(T_aI)
  [F_aII] -> MATLAB Function/7(F_aII)
  [T_aII] -> MATLAB Function/8(T_aII)

== system Furnace/Plant/Cold water from district heating ==
  Constant : Constant  Value=reg.const_F_from_DH
  Constant2 : Constant  Value=reg.const_T_from_DH
  From Workspace1 : FromWorkspace  VariableName=F_from_DH
  From Workspace2 : FromWorkspace  VariableName=T_from_DH
  Selector : Selector  InputPortWidth=2  IndexOptions=Index vector (dialog)  Indices=reg.input_type_F_from_DH  OutputSizes=1
  Selector1 : Selector  InputPortWidth=2  IndexOptions=Index vector (dialog)  Indices=reg.input_type_T_from_DH  OutputSizes=1
  Vector Concatenate : Concatenate
  Vector Concatenate1 : Concatenate
  Out1 : Outport  VectorParamsAs1DForOutWhenUnconnected=off
  Out2 : Outport  Port=2  VectorParamsAs1DForOutWhenUnconnected=off
  wires:
  From Workspace1/1 -> Vector Concatenate/2
  Constant/1 -> Vector Concatenate/1
  Constant2/1 -> Vector Concatenate1/1
  From Workspace2/1 -> Vector Concatenate1/2
  Vector Concatenate/1 -> Selector/1
  Selector/1 -> Out1/1  "F_from_DH"
  Vector Concatenate1/1 -> Selector1/1
  Selector1/1 -> Out2/1  "T_from_DH"
